simulink model "active_suspension_sim"  (Simulink 8.3)
settings: Solver=ode45  SolverMode=SingleTasking  StartTime=0.0  StopTime=10.0  RelTol=1e-3
values from neighbouring files (symbols this model uses):
  A = [[0 1 0 0 0];[-(cw+cs)/mw -ds/mw cs/mw ds/mw -1/mw];[0 0 0 1 0];[cs/mc ds/mc -cs/mc -ds/mc 1/mc];[0 0 0 0 -1/tau]]    [active_suspension_ctrl_design.m]
  B1 = [B H]    [active_suspension_ctrl_design.m]
  C = [[-1 0 1 0 0];[cs/mc ds/mc -cs/mc -ds/mc 1/mc]]    [active_suspension_ctrl_design.m]
  C1 = eye(5)    [active_suspension_ctrl_design.m]
  D1 = zeros(5,2)    [active_suspension_ctrl_design.m]
undefined symbols (not defined in the file or in its folder): K
settings Model: Creator=JonasMac  LastModifiedBy=rodralez  CovSFcnEnable=on
settings OptimizationCC: BlockReduction=off  BooleanDataType=off
settings DebuggingCC: SaveWithParameterizedLinksMsg=none  SignalResolutionControl=TryResolveAllWithWarning  SolverPrmCheckMsg=none  MultiTaskDSMMsg=warning  MultiTaskCondExecSysMsg=none  FrameProcessingCompatibilityMsg=error  StateNameClashWarn=none
settings HardwareCC: TargetUnknown=on
settings GRTTargetCC: CombineOutputUpdateFcns=on  GRTInterface=off

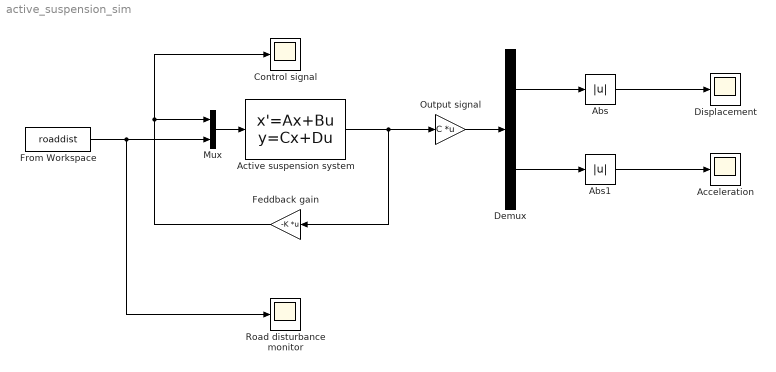
== system active_suspension_sim ==
  Abs : Abs
  Abs1 : Abs
  Acceleration : Scope
      settings: TimeRange=auto  LimitDataPoints=on  MaxDataPoints=5000  SaveToWorkspace=off  SaveName=ScopeData  YMin=0.00015  YMax=0.00196  SampleTime=-1  DataFormat=Array
  Active suspension system : StateSpace  A=A  B=B1  C=C1  D=D1
  Control signal : Scope
      settings: TimeRange=auto  LimitDataPoints=on  MaxDataPoints=5000  SaveToWorkspace=off  SaveName=ScopeData  YMin=-10  YMax=10  SampleTime=-1  DataFormat=Array
  Demux : Demux  Outputs=2
  Displacement : Scope
      settings: TimeRange=auto  LimitDataPoints=on  MaxDataPoints=5000  SaveToWorkspace=off  SaveName=ScopeData  YMin=-0.00473  YMax=0.04258  SampleTime=-1  DataFormat=Array
  Feddback gain : Gain  Gain=-K  Multiplication=Matrix(K*u)
  From Workspace : FromWorkspace  VariableName=roaddist
  Mux : Mux  Inputs=2
  Output signal : Gain  Gain=C  Multiplication=Matrix(K*u)
  Road disturbance monitor : Scope
      settings: TimeRange=auto  LimitDataPoints=on  MaxDataPoints=5000  SaveToWorkspace=off  SaveName=ScopeData  YMin=-10  YMax=10  SampleTime=-1  DataFormat=Array
  wires:
  Demux/1 -> Abs/1
  Active suspension system/1 -> Feddback gain/1, Output signal/1
  Feddback gain/1 -> Mux/1, Control signal/1
  Mux/1 -> Active suspension system/1
  Output signal/1 -> Demux/1
  Demux/2 -> Abs1/1
  From Workspace/1 -> Road disturbance monitor/1, Mux/2
  Abs/1 -> Displacement/1
  Abs1/1 -> Acceleration/1
